simulink model "COMPARISON"  (Simulink 8.6)
settings: Solver=ode45  StartTime=0.0  StopTime=2  RelTol=1e-3
settings Model: Creator=japerez  LastModifiedBy=d.alazard
settings DataIOCC: SignalLoggingSaveFormat=Dataset
settings OptimizationCC: ExpressionDepthLimit=128
settings DebuggingCC: UnderspecifiedInitializationDetection=Simplified  MergeDetectMultiDrivingBlocksExec=error  FcnCallInpInsideContextMsg=EnableAllAsError  StateNameClashWarn=none
settings GRTTargetCC: CombineOutputUpdateFcns=on  GRTInterface=off
settings ConfigComp: CovSFcnEnable=off

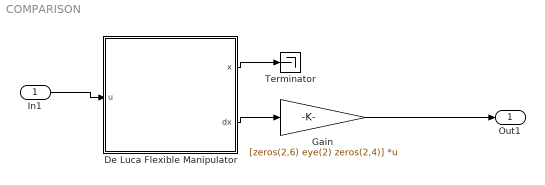
== system COMPARISON ==
  In1 : Inport  PortDimensions=2
  De Luca Flexible Manipulator : Subsystem
  Gain : Gain  Gain=[zeros(2,6) eye(2) zeros(2,4)]  Multiplication=Matrix(K*u) (u vector)
  Terminator : Terminator
  Out1 : Outport
  wires:
  In1/1 -> De Luca Flexible Manipulator/1(u)
  De Luca Flexible Manipulator/1(x) -> Terminator/1
  De Luca Flexible Manipulator/2(dx) -> Gain/1
  Gain/1 -> Out1/1

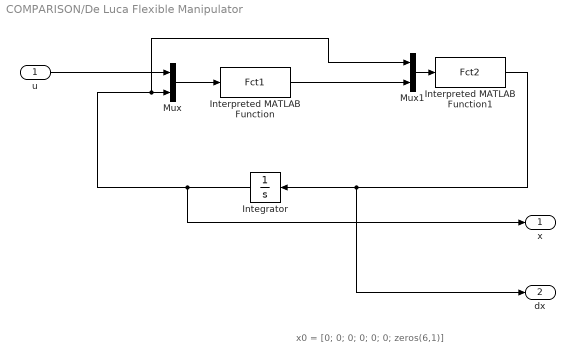
== system COMPARISON/De Luca Flexible Manipulator ==
  note: x0 = [0; 0; 0; 0; 0; 0; zeros(6,1)]
  u : Inport  PortDimensions=2
  Integrator : Integrator  InitialCondition=[0; 0; 0; 0; 0; 0; zeros(6,1)]
  Interpreted MATLAB Function : MATLABFcn  MATLABFcn=Fct1  OutputDimensions=12
  Interpreted MATLAB Function1 : MATLABFcn  MATLABFcn=Fct2  OutputDimensions=12
  Mux : Mux  Inputs=[2 12]
  Mux1 : Mux  Inputs=[12 12]
  x : Outport  PortDimensions=12
  dx : Outport  Port=2  PortDimensions=12
  wires:
  u/1 -> Mux/1
  Interpreted MATLAB Function1/1 -> dx/1, Integrator/1
  Mux/1 -> Interpreted MATLAB Function/1
  Interpreted MATLAB Function/1 -> Mux1/2
  Integrator/1 -> x/1, Mux1/1, Mux/2
  Mux1/1 -> Interpreted MATLAB Function1/1
